simulink model "ADFT"  (R2020b)
settings: Solver=VariableStepAuto  StartTime=0.0  StopTime=1024  RelTol=1e-3
libraries: xbsIndex_r4 x129
settings Model: Creator=666sk  LastModifiedBy=666sk

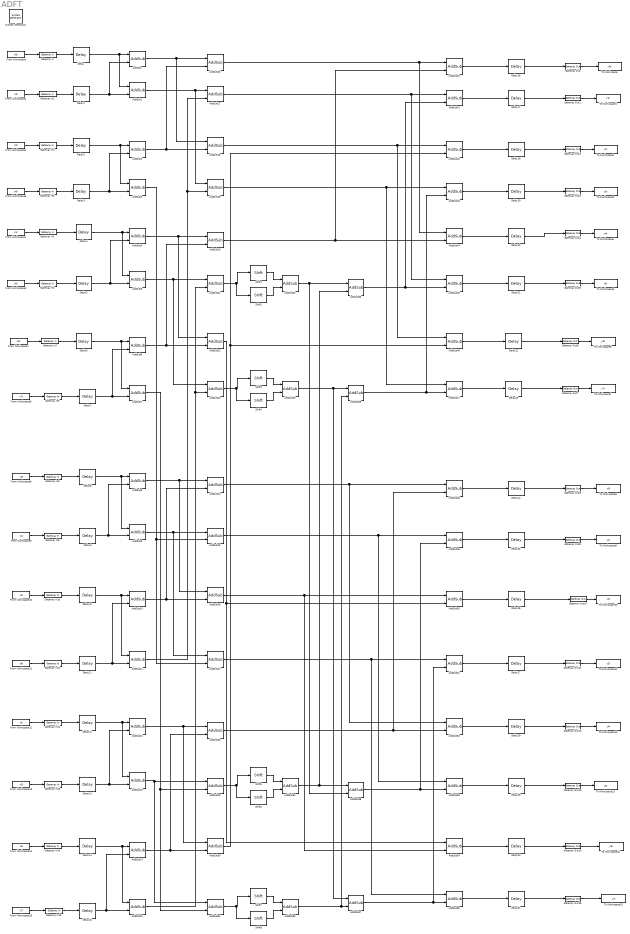
== system ADFT ==
  " System Generator" : xbsIndex_r4/ System Generator  Tag=genX  xilinxfamily=artix7  part=xc7a100t  speed=-1  package=csg324  synthesis_tool=Vivado  clock_wrapper=Clock Enables  directory=C:/Users/666sk/Desktop  proj_type=Vivado  Synth_file=Vivado Synthesis Defaults  Impl_file=Vivado Implementation Defaults  testbench=off  simulink_period=1  sysclk_period=20  dcm_input_clock_period=10  incr_netlist=off  trim_vbits=Everywhere in SubSystem  dbl_ovrd=According to Block Masks  core_generation=According to Block Masks  run_coregen=off  deprecated_control=off  eval_field=0  block_type=sysgen
  AddSub{,2,4,6,8,10,12,14,16..17,20..21,24,27..28,31..37,40..42,47..49,54..55} (30 alike) : xbsIndex_r4/AddSub  mode=Addition  use_carryin=off  use_carryout=off  en=off  latency=0  precision=User Defined  arith_type="Signed  (2's comp)"  n_bits=W  bin_pt=D  quantization="Round  (unbiased: +/- Inf)"  overflow=Saturate  use_behavioral_HDL=off  hw_selection=Fabric  pipelined=off  dbl_ovrd=off  block_type=addsub
  AddSub{1,3,5,7,9,11,13,15,18..19,22..23,25..26,29..30,38..39,43..46,50..53} (26 alike) : xbsIndex_r4/AddSub  mode=Subtraction  use_carryin=off  use_carryout=off  en=off  latency=0  precision=User Defined  arith_type="Signed  (2's comp)"  n_bits=W  bin_pt=D  quantization="Round  (unbiased: +/- Inf)"  overflow=Saturate  use_behavioral_HDL=off  hw_selection=Fabric  pipelined=off  dbl_ovrd=off  block_type=addsub
  Delay{,1..31} (32 alike) : xbsIndex_r4/Delay  rst=off  infoeditControl=Selection of Reset will increase slice count due to use of real FFs and instead of SRLs  en=off  latency=1  reg_retiming=off  dbl_ovrd=off  block_type=delay
  From Workspace : FromWorkspace  VariableName=v0r
  From Workspace1 : FromWorkspace  VariableName=v1r
  From Workspace10 : FromWorkspace  VariableName=v2i
  From Workspace11 : FromWorkspace  VariableName=v6i
  From Workspace12 : FromWorkspace  VariableName=v1i
  From Workspace13 : FromWorkspace  VariableName=v5i
  From Workspace14 : FromWorkspace  VariableName=v3i
  From Workspace15 : FromWorkspace  VariableName=v7i
  From Workspace2 : FromWorkspace  VariableName=v4r
  From Workspace3 : FromWorkspace  VariableName=v5r
  From Workspace4 : FromWorkspace  VariableName=v2r
  From Workspace5 : FromWorkspace  VariableName=v7r
  From Workspace6 : FromWorkspace  VariableName=v6r
  From Workspace7 : FromWorkspace  VariableName=v3r
  From Workspace8 : FromWorkspace  VariableName=v0i
  From Workspace9 : FromWorkspace  VariableName=v4i
  Gateway In{,1..15} (16 alike) : xbsIndex_r4/Gateway In  gui_display_data_type=Fixed-point  arith_type="Signed  (2's comp)"  n_bits=16  bin_pt=14  preci_type=Single  exp_width=8  frac_width=24  rows=1  columns=1  quantization="Round  (unbiased: +/- Inf)"  overflow=Saturate  period=1  UseAsADC=off  ADCChannel='1'  interface=None  automatic_assignment=on  address_offset=hex2dec('00')  intf_name=''  intf_description=''  default_value=0  timing_constraint=None  locs_specified=off  LOCs={}  io_standard={}  inherit_from_input=off  hdl_port=on  dbl_ovrd=off  block_type=gatewayin
  Gateway Out{,1..15} (16 alike) : xbsIndex_r4/Gateway Out  inherit_from_input=off  hdl_port=on  rows=1  columns=1  UseAsDAC=off  DACChannel='1'  interface=None  automatic_assignment=on  address_offset=hex2dec('00')  intf_name=''  intf_description=''  timing_constraint=None  locs_specified=off  LOCs={}  io_standard={}  block_type=gatewayout
  Shift{1,3,5,7} (4 alike) : xbsIndex_r4/Shift  shift_dir=Right  shift_bits=1  en=off  latency=0  precision=Full  arith_type="Signed  (2's comp)"  n_bits=16  bin_pt=14  quantization=Truncate  overflow=Wrap  dbl_ovrd=off  block_type=shift
  Shift{2,4,6,8} (4 alike) : xbsIndex_r4/Shift  shift_dir=Right  shift_bits=2  en=off  latency=0  precision=Full  arith_type="Signed  (2's comp)"  n_bits=16  bin_pt=14  quantization=Truncate  overflow=Wrap  dbl_ovrd=off  block_type=shift
  To Workspace : ToWorkspace  VariableName=y0r  SaveFormat=Timeseries  SampleTime=-1
  To Workspace1 : ToWorkspace  VariableName=y1r  SaveFormat=Timeseries  SampleTime=-1
  To Workspace10 : ToWorkspace  VariableName=y2i  SaveFormat=Timeseries  SampleTime=-1
  To Workspace11 : ToWorkspace  VariableName=y3i  SaveFormat=Timeseries  SampleTime=-1
  To Workspace12 : ToWorkspace  VariableName=y4i  SaveFormat=Timeseries  SampleTime=-1
  To Workspace13 : ToWorkspace  VariableName=y5i  SaveFormat=Timeseries  SampleTime=-1
  To Workspace14 : ToWorkspace  VariableName=y6i  SaveFormat=Timeseries  SampleTime=-1
  To Workspace15 : ToWorkspace  VariableName=y7i  SaveFormat=Timeseries  SampleTime=-1
  To Workspace2 : ToWorkspace  VariableName=y2r  SaveFormat=Timeseries  SampleTime=-1
  To Workspace3 : ToWorkspace  VariableName=y3r  SaveFormat=Timeseries  SampleTime=-1
  To Workspace4 : ToWorkspace  VariableName=y4r  SaveFormat=Timeseries  SampleTime=-1
  To Workspace5 : ToWorkspace  VariableName=y5r  SaveFormat=Timeseries  SampleTime=-1
  To Workspace6 : ToWorkspace  VariableName=y6r  SaveFormat=Timeseries  SampleTime=-1
  To Workspace7 : ToWorkspace  VariableName=y7r  SaveFormat=Timeseries  SampleTime=-1
  To Workspace8 : ToWorkspace  VariableName=y0i  SaveFormat=Timeseries  SampleTime=-1
  To Workspace9 : ToWorkspace  VariableName=y1i  SaveFormat=Timeseries  SampleTime=-1
  wires:
  From Workspace1/1 -> Gateway In1/1
  From Workspace2/1 -> Gateway In2/1
  From Workspace3/1 -> Gateway In3/1
  From Workspace4/1 -> Gateway In4/1
  From Workspace5/1 -> Gateway In5/1
  From Workspace6/1 -> Gateway In6/1
  From Workspace7/1 -> Gateway In7/1
  Gateway In2/1 -> Delay1/1
  Gateway In/1 -> Delay/1
  Gateway In4/1 -> Delay2/1
  Gateway In6/1 -> Delay3/1
  Gateway In1/1 -> Delay4/1
  Gateway In3/1 -> Delay5/1
  Gateway In7/1 -> Delay6/1
  Gateway In5/1 -> Delay7/1
  Delay/1 -> AddSub1/1, AddSub/1
  Delay1/1 -> AddSub1/2, AddSub/2
  From Workspace8/1 -> Gateway In8/1
  Gateway In8/1 -> Delay8/1
  From Workspace9/1 -> Gateway In9/1
  Gateway In9/1 -> Delay9/1
  From Workspace10/1 -> Gateway In10/1
  Gateway In10/1 -> Delay10/1
  From Workspace11/1 -> Gateway In11/1
  Gateway In11/1 -> Delay11/1
  From Workspace12/1 -> Gateway In12/1
  Gateway In12/1 -> Delay12/1
  From Workspace13/1 -> Gateway In13/1
  Gateway In13/1 -> Delay13/1
  From Workspace14/1 -> Gateway In14/1
  Gateway In14/1 -> Delay14/1
  From Workspace15/1 -> Gateway In15/1
  Gateway In15/1 -> Delay15/1
  Delay2/1 -> AddSub3/1, AddSub2/1
  Delay3/1 -> AddSub3/2, AddSub2/2
  Delay4/1 -> AddSub5/1, AddSub4/1
  Delay5/1 -> AddSub5/2, AddSub4/2
  Delay6/1 -> AddSub7/1, AddSub6/1
  Delay7/1 -> AddSub7/2, AddSub6/2
  Delay8/1 -> AddSub9/1, AddSub8/1
  Delay9/1 -> AddSub9/2, AddSub8/2
  Delay10/1 -> AddSub11/1, AddSub10/1
  Delay11/1 -> AddSub11/2, AddSub10/2
  Delay13/1 -> AddSub12/2, AddSub13/2
  Delay12/1 -> AddSub13/1, AddSub12/1
  Delay15/1 -> AddSub15/2, AddSub14/2
  Delay14/1 -> AddSub15/1, AddSub14/1
  AddSub/1 -> AddSub18/1, AddSub16/1
  AddSub2/1 -> AddSub18/2, AddSub16/2
  AddSub1/1 -> AddSub19/1, AddSub17/1
  AddSub11/1 -> AddSub19/2, AddSub17/2
  AddSub4/1 -> AddSub22/1, AddSub20/1
  AddSub6/1 -> AddSub22/2, AddSub20/2
  AddSub5/1 -> AddSub23/1, AddSub21/1
  AddSub15/1 -> AddSub23/2, AddSub21/2
  AddSub7/1 -> AddSub31/2, AddSub29/2
  AddSub8/1 -> AddSub26/1, AddSub24/1
  AddSub10/1 -> AddSub26/2, AddSub24/2
  AddSub9/1 -> AddSub27/1, AddSub25/1
  AddSub3/1 -> AddSub27/2, AddSub25/2
  AddSub12/1 -> AddSub30/1, AddSub28/1
  AddSub14/1 -> AddSub28/2, AddSub30/2
  AddSub13/1 -> AddSub31/1, AddSub29/1
  Shift1/1 -> AddSub32/1
  Shift2/1 -> AddSub32/2
  AddSub21/1 -> Shift2/1, Shift1/1
  Shift3/1 -> AddSub33/1
  Shift4/1 -> AddSub33/2
  AddSub23/1 -> Shift4/1, Shift3/1
  Shift5/1 -> AddSub34/1
  Shift6/1 -> AddSub34/2
  AddSub29/1 -> Shift6/1, Shift5/1
  Shift7/1 -> AddSub35/1
  Shift8/1 -> AddSub35/2
  AddSub31/1 -> Shift8/1, Shift7/1
  AddSub32/1 -> AddSub38/2, AddSub36/1
  AddSub34/1 -> AddSub38/1, AddSub36/2
  AddSub35/1 -> AddSub39/2, AddSub37/2
  AddSub33/1 -> AddSub39/1, AddSub37/1
  AddSub16/1 -> AddSub44/1, AddSub40/1
  AddSub20/1 -> AddSub44/2, AddSub40/2
  AddSub17/1 -> AddSub45/1, AddSub41/1
  AddSub36/1 -> AddSub45/2, AddSub41/2
  AddSub18/1 -> AddSub46/1, AddSub42/1
  AddSub30/1 -> AddSub46/2, AddSub42/2
  AddSub19/1 -> AddSub47/1, AddSub43/1
  AddSub39/1 -> AddSub47/2, AddSub43/2
  AddSub24/1 -> AddSub52/1, AddSub48/1
  AddSub28/1 -> AddSub52/2, AddSub48/2
  AddSub25/1 -> AddSub53/1, AddSub49/1
  AddSub38/1 -> AddSub53/2, AddSub49/2
  AddSub26/1 -> AddSub54/2, AddSub50/1
  AddSub22/1 -> AddSub54/1, AddSub50/2
  AddSub27/1 -> AddSub55/1, AddSub51/1
  AddSub37/1 -> AddSub55/2, AddSub51/2
  Delay16/1 -> Gateway Out/1
  AddSub40/1 -> Delay16/1
  Delay17/1 -> Gateway Out1/1
  AddSub41/1 -> Delay17/1
  Delay18/1 -> Gateway Out2/1
  Gateway Out2/1 -> To Workspace2/1
  AddSub42/1 -> Delay18/1
  Delay19/1 -> Gateway Out3/1
  Gateway Out3/1 -> To Workspace3/1
  AddSub43/1 -> Delay19/1
  Delay20/1 -> Gateway Out4/1
  Gateway Out4/1 -> To Workspace4/1
  AddSub44/1 -> Delay20/1
  Delay21/1 -> Gateway Out5/1
  Gateway Out5/1 -> To Workspace5/1
  AddSub45/1 -> Delay21/1
  Delay22/1 -> Gateway Out6/1
  Gateway Out6/1 -> To Workspace6/1
  AddSub46/1 -> Delay22/1
  Delay23/1 -> Gateway Out7/1
  Gateway Out7/1 -> To Workspace7/1
  AddSub47/1 -> Delay23/1
  Delay24/1 -> Gateway Out8/1
  Gateway Out8/1 -> To Workspace8/1
  AddSub48/1 -> Delay24/1
  Delay25/1 -> Gateway Out9/1
  Gateway Out9/1 -> To Workspace9/1
  AddSub49/1 -> Delay25/1
  Delay26/1 -> Gateway Out10/1
  AddSub50/1 -> Delay26/1
  Delay27/1 -> Gateway Out11/1
  Gateway Out11/1 -> To Workspace11/1
  AddSub51/1 -> Delay27/1
  Delay28/1 -> Gateway Out12/1
  Gateway Out12/1 -> To Workspace12/1
  AddSub52/1 -> Delay28/1
  Delay29/1 -> Gateway Out13/1
  Gateway Out13/1 -> To Workspace13/1
  AddSub53/1 -> Delay29/1
  Delay30/1 -> Gateway Out14/1
  AddSub54/1 -> Delay30/1
  Delay31/1 -> Gateway Out15/1
  AddSub55/1 -> Delay31/1
  Gateway Out/1 -> To Workspace/1
  Gateway Out1/1 -> To Workspace1/1
  Gateway Out10/1 -> To Workspace10/1
  Gateway Out14/1 -> To Workspace14/1
  Gateway Out15/1 -> To Workspace15/1
  From Workspace/1 -> Gateway In/1
